simulink model "EMA_model"  (R2023b)
settings: Solver=VariableStepAuto  StartTime=0.0  StopTime=10.0  RelTol=1e-3
undefined symbols (not defined in the file): Bd, F_load, K, Ke, Kf, Kt, L, m, R, Vdc
libraries: simulink x1, slpidlib x1
settings Model: Creator=lenovo  LastModifiedBy=lenovo

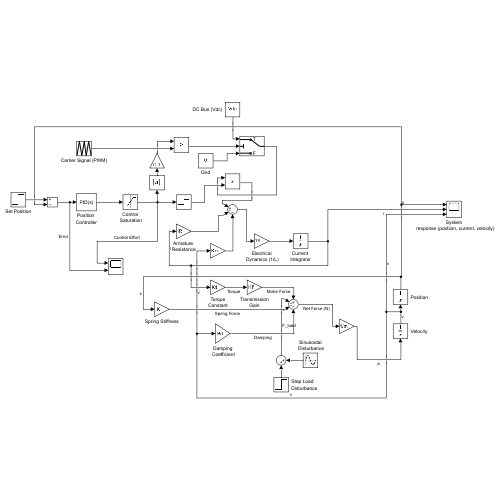
[thumbnail: Simulink's stored preview of the top-level diagram]
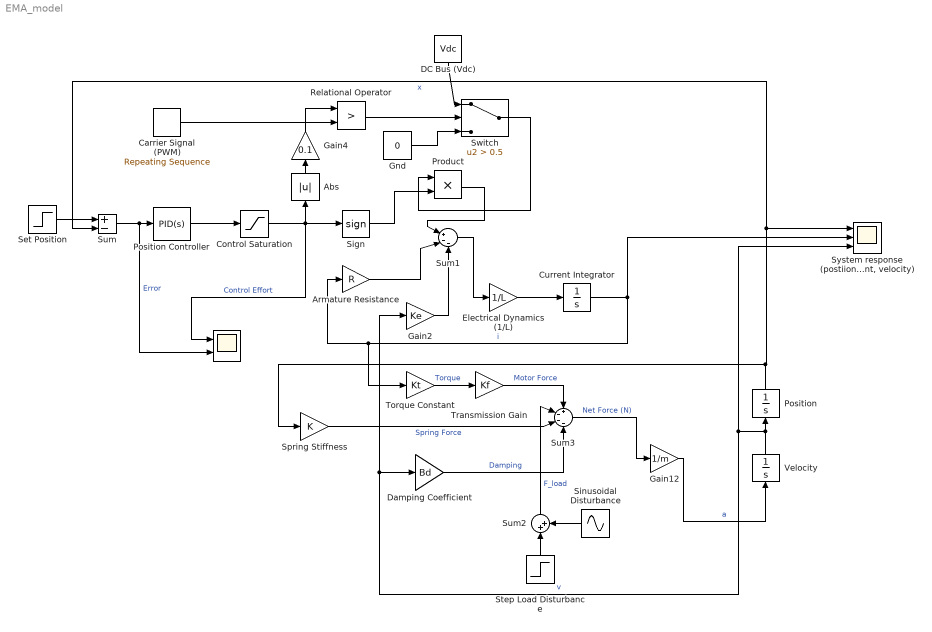
== system EMA_model ==
  " " : Scope  NumInputPorts=2
  Abs : Abs  SaturateOnIntegerOverflow=off
  Armature Resistance : Gain  Gain=R
  Carrier Signal (PWM) : simulink/Sources/Repeating Sequence  rep_seq_t=[0 0.00005 0.0001]  rep_seq_y=[0 1 0]
  Control Saturation : Saturate  UpperLimit=10  LowerLimit=-10
  Current Integrator : Integrator
  DC Bus (Vdc) : Constant  Value=Vdc
  Damping Coefficient : Gain  Gain=Bd
  Electrical Dynamics (1/L) : Gain  Gain=1/L
  Gain12 : Gain  Gain=1/m
  Gain2 : Gain  Gain=Ke
  Gain4 : Gain  Gain=0.1
  Gnd : Constant  Value=0
  Position : Integrator
  Position Controller : slpidlib/PID Controller  Controller=PID  Form=Parallel  TimeDomain=Continuous-time  UseExternalTs=off  SampleTime=-1  IntegratorMethod=Forward Euler  FilterMethod=Forward Euler  ControllerParametersSource=internal  P=28.2455993595637  I=8.2169735690655  UseKiTs=off  D=10.11075197099066  N=731.766951260832  UseFilter=on  TunerSelectOption=Transfer Function Based (PID Tuner App)  InitialConditionSource=internal  InitialConditionForIntegrator=0  InitialConditionForFilter=0  DifferentiatorICPrevScaledInput=0  ExternalReset=none  TrackingMode=off  Kt=1  LimitOutput=off  SatLimitsSource=internal  UpperSaturationLimit=inf  LowerSaturationLimit=-inf  LinearizeAsGain=on  AntiWindupMode=none  Kb=1  LimitIntegrator=off  UpperIntegratorSaturationLimit=inf  LowerIntegratorSaturationLimit=-inf  POutMin=[]  POutMax=[]  IOutMin=[]  IOutMax=[]  DOutMin=[]  DOutMax=[]  NOutMin=[]  NOutMax=[]  SumOutMin=[]  SumOutMax=[]  SaturationOutMin=[]  SaturationOutMax=[]  PParamMin=[]  PParamMax=[]  IParamMin=[]  IParamMax=[]  DParamMin=[]  DParamMax=[]  NParamMin=[]  NParamMax=[]  KbParamMin=[]  KbParamMax=[]  KtParamMin=[]  KtParamMax=[]  KbOutMin=[]  KbOutMax=[]  KtOutMin=[]  KtOutMax=[]  IntegratorOutMin=[]  IntegratorOutMax=[]  FilterOutMin=[]  FilterOutMax=[]  SumI1OutMin=[]  SumI1OutMax=[]  SumI2OutMin=[]  SumI2OutMax=[]  SumI3OutMin=[]  SumI3OutMax=[]  SumI4OutMin=[]  SumI4OutMax=[]  SumDOutMin=[]  SumDOutMax=[]  DifferentiatorOutMin=[]  DifferentiatorOutMax=[]  FilterDiffOutCoefMin=[]  FilterDiffOutCoefMax=[]  ReciprocalOutMin=[]  ReciprocalOutMax=[]  SumDenOutMin=[]  SumDenOutMax=[]  SumNumOutMin=[]  SumNumOutMax=[]  DivideOutMin=[]  DivideOutMax=[]  UdiffTsProdOutMin=[]  UdiffTsProdOutMax=[]  NTsProdOutMin=[]  NTsProdOutMax=[]  UintegralTsProdOutMin=[]  UintegralTsProdOutMax=[]  UngainTsProdOutMin=[]  UngainTsProdOutMax=[]  ClampingZeroOutDataTypeStr=Inherit: Inherit via back propagation  ClampingZeroOutMin=[]  ClampingZeroOutMax=[]  FilterDenConstantOutDataTypeStr=Inherit: Inherit via back propagation  FilterDenConstantOutMin=[]  FilterDenConstantOutMax=[]  PCopyOutDataTypeStr=Inherit: Inherit via back propagation  PCopyOutMin=[]  PCopyOutMax=[]  NCopyOutDataTypeStr=Inherit: Inherit via back propagation  NCopyOutMin=[]  NCopyOutMax=[]  IntegratorContinuousStateAttributes=''  IntegratorStateMustResolveToSignalObject=off  IntegratorRTWStateStorageClass=Auto  FilterContinuousStateAttributes=''  FilterStateMustResolveToSignalObject=off  FilterRTWStateStorageClass=Auto  ParallelPVariant=InternalParameters  IdealPVariant=Disabled  IVariant=InternalParameters  DVariant=InternalParameters  IntegratorVariant=Continuous  SatVariant=Disabled  AWVariant=Passthrough  PCopyVariant=Disabled  TRVariant=Disabled  FdbkBlocksVariant=Forward  IdealPFdbkVariant=Disabled  SatFdbkVariant=Disabled  DerivativeFilterVariant=ContFilter  NVariant=InternalParameters  NCopyVariant=Disabled  FilterICVariant=InternalICsFilter  IntegratorICVariant=InternalICs  ExternalResetVariant=Disabled  TRSumVariant=Passthrough  SumFdbkVariant=Disabled  SumVariant=Sum_PID  TsampFilterVariant=InternalTs  TsampNgainVariant=Passthrough  TsampIntegralVariant=Disabled_SignalSpec  ExternalSaturationOutDataTypeStr=Inherit: Same as second input
  Product : Product
  Relational Operator : RelationalOperator  Operator=>  OutDataTypeStr=boolean  RndMeth=Simplest  InputSameDT=off
  Set Position : Step  Time=0  SampleTime=0
  Sign : Signum
  Sinusoidal Disturbance : Sin  Amplitude=8  Frequency=2  SampleTime=0
  Spring Stiffness : Gain  Gain=K
  Step Load Disturbance : Step  After=F_load  SampleTime=0
  Sum : Sum  Inputs=+-
  Sum1 : Sum  Inputs=|+--
  Sum2 : Sum  Inputs=|++
  Sum3 : Sum  Inputs=+---
  Switch : Switch  Criteria=u2 > Threshold  Threshold=0.5  SaturateOnIntegerOverflow=off  InputSameDT=off
  "System response (postiion, current, velocity)" : Scope  NumInputPorts=3
  Torque Constant : Gain  Gain=Kt
  Transmission Gain : Gain  Gain=Kf
  Velocity : Integrator
  wires:
  Set Position/1 -> Sum/1
  Armature Resistance/1 -> Sum1/2
  Current Integrator/1 -> Torque Constant/1, Armature Resistance/1, "System response (postiion, current, velocity)"/2  "i"
  Gain2/1 -> Sum1/3
  Sum1/1 -> Electrical Dynamics (1/L)/1
  Electrical Dynamics (1/L)/1 -> Current Integrator/1
  Relational Operator/1 -> Switch/2
  DC Bus (Vdc)/1 -> Switch/1
  Gnd/1 -> Switch/3
  Carrier Signal (PWM)/1 -> Relational Operator/2
  Sum/1 -> " "/2, Position Controller/1  "Error"
  Gain4/1 -> Relational Operator/1
  Control Saturation/1 -> " "/1, Sign/1, Abs/1  "Control Effort"
  Abs/1 -> Gain4/1
  Sign/1 -> Product/2
  Switch/1 -> Product/1
  Product/1 -> Sum1/1
  Position/1 -> Sum/2, "System response (postiion, current, velocity)"/1, Spring Stiffness/1  "x"
  Position Controller/1 -> Control Saturation/1
  Torque Constant/1 -> Transmission Gain/1  "Torque"
  Transmission Gain/1 -> Sum3/1  "Motor Force"
  Damping Coefficient/1 -> Sum3/4  "Damping"
  Spring Stiffness/1 -> Sum3/3  "Spring Force"
  Sum3/1 -> Gain12/1  "Net Force (N)"
  Gain12/1 -> Velocity/1  "a"
  Velocity/1 -> Damping Coefficient/1, Gain2/1, "System response (postiion, current, velocity)"/3, Position/1  "v"
  Step Load Disturbance/1 -> Sum2/1
  Sinusoidal Disturbance/1 -> Sum2/2
  Sum2/1 -> Sum3/2  "F_load"
